simulink model "Motor_Position"  (R2020b)
settings: Solver=VariableStepAuto  StartTime=0.0  StopTime=10.0  RelTol=1e-3
values from neighbouring files (symbols this model uses):
  b = 3.5077E-6    [Problem4_data.sldd]
  J = 3.2284E-6    [Problem4_data.sldd]
  Ke = 0.0274    [Problem4_data.sldd]
  Kt = 0.0274    [Problem4_data.sldd]
  L = 2.75E-6    [Problem4_data.sldd]
  R = 4.0    [Problem4_data.sldd]
settings Model: DataDictionary=Problem4_data.sldd  Creator=ASUS  LastModifiedBy=ASUS
settings DataIOCC: SaveOutput=off  SaveTime=off

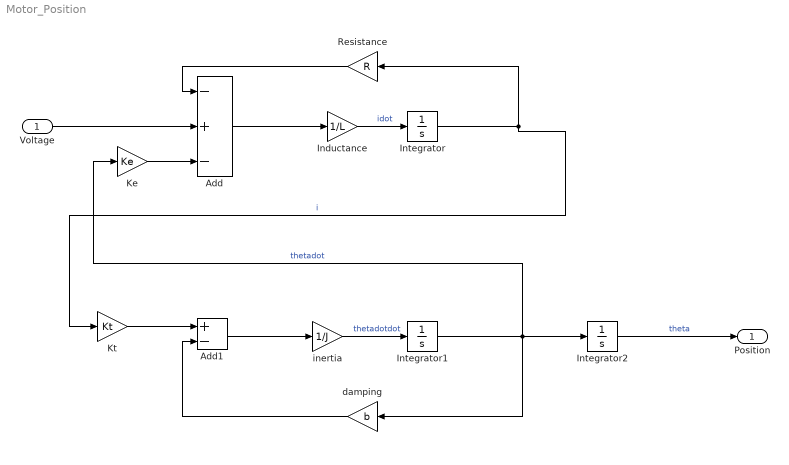
== system Motor_Position ==
  Voltage : Inport  OutDataTypeStr=double  PortDimensions=1
  Add : Sum  Inputs=-+-
  Add1 : Sum  Inputs=+-
  Inductance : Gain  Gain=1/L
  Integrator : Integrator
  Integrator1 : Integrator
  Integrator2 : Integrator
  Ke : Gain  Gain=Ke
  Kt : Gain  Gain=Kt
  Resistance : Gain  Gain=R
  damping : Gain  Gain=b
  inertia : Gain  Gain=1/J
  Position : Outport  OutDataTypeStr=double  PortDimensions=1  SampleTime=0
  wires:
  Add/1 -> Inductance/1
  Integrator2/1 -> Position/1  "theta"
  Kt/1 -> Add1/1
  Add1/1 -> inertia/1
  Inductance/1 -> Integrator/1  "idot"
  Resistance/1 -> Add/1
  damping/1 -> Add1/2
  Integrator/1 -> Resistance/1, Kt/1  "i"
  inertia/1 -> Integrator1/1  "thetadotdot"
  Integrator1/1 -> Integrator2/1, damping/1, Ke/1  "thetadot"
  Ke/1 -> Add/3
  Voltage/1 -> Add/2
